simulink model "SlidingMode_HW3_DynamicSMC"  (R2021a)
settings: Solver=VariableStepAuto  StartTime=0.0  StopTime=10.0  RelTol=1e-3
settings Model: Creator=kiankhaneghahi  LastModifiedBy=kiankhaneghahi
settings SolverCC: ZeroCrossAlgorithm=Adaptive
settings DebuggingCC: IgnoredZcDiagnostic=none

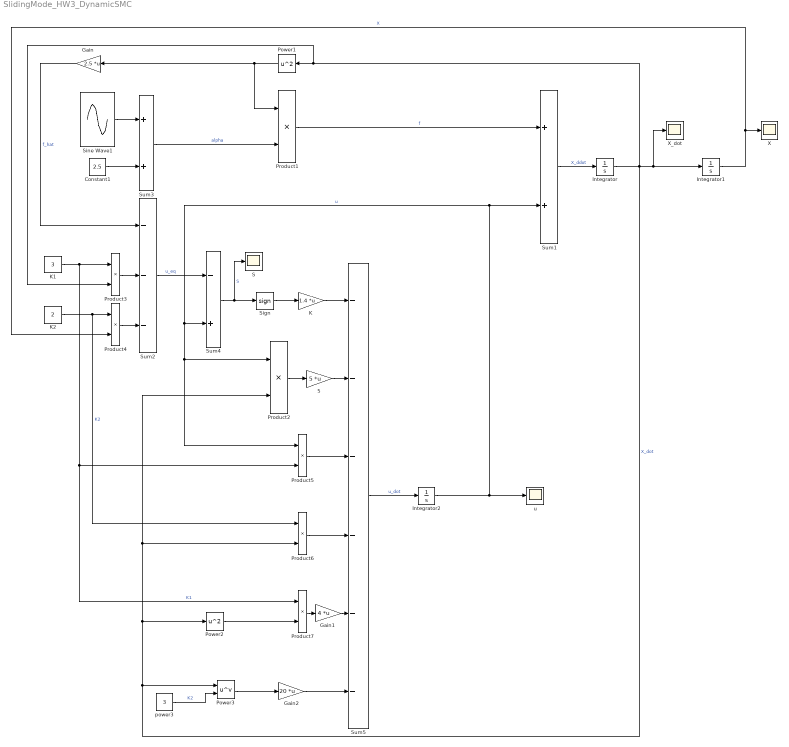
== system SlidingMode_HW3_DynamicSMC ==
  5 : Gain  Gain=5  Multiplication=Matrix(K*u)
  Constant1 : Constant  Value=2.5
  Gain : Gain  Gain=2.5  Multiplication=Matrix(K*u)
  Gain1 : Gain  Gain=4  Multiplication=Matrix(K*u)
  Gain2 : Gain  Gain=20  Multiplication=Matrix(K*u)
  Integrator : Integrator  InitialCondition=1
  Integrator1 : Integrator  InitialCondition=2
  Integrator2 : Integrator
  K : Gain  Gain=1.4  Multiplication=Matrix(K*u)
  K1 : Constant  Value=3
  K2 : Constant  Value=2
  Power1 : Math  Operator=square  SaturateOnIntegerOverflow=on
  Power2 : Math  Operator=square  SaturateOnIntegerOverflow=on
  Power3 : Math  Operator=pow  SaturateOnIntegerOverflow=on
  Product{1..7} (7 alike) : Product
  S : Scope
  Sign : Signum
  Sine Wave1 : Sin  Amplitude=1.5  SampleTime=0
  Sum1 : Sum
  Sum2 : Sum  Inputs=---
  Sum3 : Sum
  Sum4 : Sum  Inputs=-+
  Sum5 : Sum  Inputs=------
  X : Scope
  X_dot : Scope
  power3 : Constant  Value=3
  u : Scope
  wires:
  Sum3/1 -> Product1/2  "alpha"
  Constant1/1 -> Sum3/2
  Sine Wave1/1 -> Sum3/1
  Sum1/1 -> Integrator/1  "X_ddot"
  Integrator/1 -> Power3/1, Power2/1, Product6/2, Product2/2, Power1/1, Product3/2, X_dot/1, Integrator1/1  "X_dot"
  Integrator1/1 -> X/1, Product4/2  "X"
  Product1/1 -> Sum1/1  "f"
  Power1/1 -> Gain/1, Product1/1
  Gain/1 -> Sum2/1  "f_hat"
  Product3/1 -> Sum2/2
  Product4/1 -> Sum2/3
  Sum2/1 -> Sum4/1  "u_eq"
  Sum4/1 -> S/1, Sign/1  "S"
  Sign/1 -> K/1
  K/1 -> Sum5/1
  Sum5/1 -> Integrator2/1  "u_dot"
  Integrator2/1 -> Sum1/2, Product2/1, Product5/1, Sum4/2, u/1  "u"
  Product2/1 -> 5/1
  5/1 -> Sum5/2
  K1/1 -> Product7/1, Product5/2, Product3/1  "K1"
  K2/1 -> Product6/1, Product4/1  "K2"
  Product5/1 -> Sum5/3
  Product6/1 -> Sum5/4
  Product7/1 -> Gain1/1
  Gain1/1 -> Sum5/5
  Power2/1 -> Product7/2
  Power3/1 -> Gain2/1
  power3/1 -> Power3/2  "K2"
  Gain2/1 -> Sum5/6
